simulink model "Earth_Moon"  (R2024a)
settings: Solver=VariableStepAuto  StartTime=0.0  StopTime=2419200  RelTol=1e-3
values from neighbouring files (symbols this model uses):
  G = 6.674e-11    [L_points.m]    (also in Lab3_Driver.m; Lab5.m; Lab8.m; LagrangePoints.m = 6.67408e-11)
  mE = 5.97219e24    (= 5.97219e+24)    [L_points.m]    (also in Lab5.m; Lab8.m; Presentation_Circular.m; Presentation_HaloOrbit.m)
  mM = 7.349e22    (= 7.349e+22)    [L_points.m]    (also in Lab5.m; Lab8.m; Presentation_Circular.m = plot3(OM(mid,1)/1000,OM(mid,2)/1000,OM(mid,3)/1000,Marker="o; Presentation_HaloOrbit.m)
  posE = [3.034529801433376E+03 -3.340359653273315E+03 -1.939037192252903E+03]*1000    [L_points.m]    (also in Lab5.m = [-xE 0 0]; Lab8.m = [-xE 0 0]; Presentation_Circular.m = [-xE 0 0]; Presentation_HaloOrbit.m = [-xE 0 0])
  posM = [-2.467089971416006E+05 2.715731378752839E+05 1.576448255327776E+05]*1000    [L_points.m]    (also in Lab5.m = [xM 0 0]; Lab8.m = [xM 0 0]; Presentation_Circular.m = [xM 0 0]; Presentation_HaloOrbit.m = [xM 0 0])
  velE = [9.245683416082787E-03 6.608382937807280E-03 2.954691314042687E-03]*1000    [L_points.m]    (also in Lab5.m = [0 -vE 0]; Lab8.m = [0 -vE 0]; Presentation_Circular.m = [0 -vE 0]; Presentation_HaloOrbit.m = [0 -vE 0])
  velM = [-7.516793153236040E-01 -5.372652878689789E-01 -2.402180827507927E-01]*1000    [L_points.m]    (also in Lab5.m = [0 vM 0]; Lab8.m = [0 vM 0]; Presentation_Circular.m = [0 vM 0]; Presentation_HaloOrbit.m = [0 vM 0])
settings Model: Creator=sgtjake2  LastModifiedBy=sgtjake2

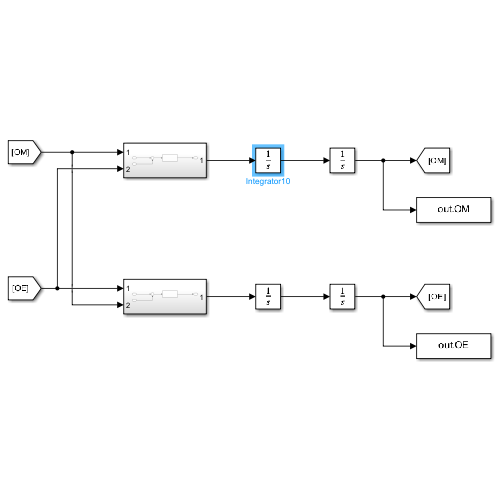
[thumbnail: Simulink's stored preview of the top-level diagram]
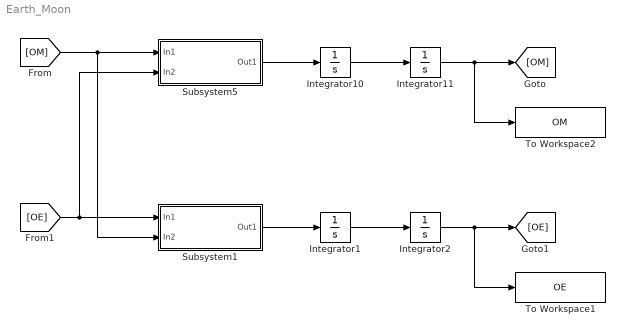
== system Earth_Moon ==
  Integrator1 : Integrator  InitialCondition=velE
  Integrator10 : Integrator  InitialCondition=velM
  Integrator11 : Integrator  InitialCondition=posM
  Integrator2 : Integrator  InitialCondition=posE
  Subsystem1 : Subsystem
  Subsystem5 : Subsystem
  To Workspace1 : ToWorkspace  VariableName=OE  SaveFormat=Timeseries  SampleTime=-1
  To Workspace2 : ToWorkspace  VariableName=OM  SaveFormat=Timeseries  SampleTime=-1
  wires:
  Integrator11/1 -> To Workspace2/1, [OM]
  [OM] -> Subsystem1/2(In2), Subsystem5/1(In1)
  Integrator10/1 -> Integrator11/1
  Integrator2/1 -> To Workspace1/1, [OE]
  [OE] -> Subsystem1/1(In1), Subsystem5/2(In2)
  Integrator1/1 -> Integrator2/1
  Subsystem5/1(Out1) -> Integrator10/1
  Subsystem1/1(Out1) -> Integrator1/1

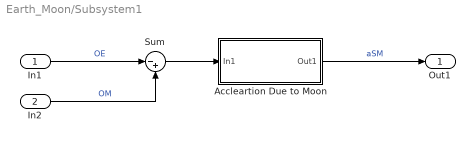
== system Earth_Moon/Subsystem1 ==
  In1 : Inport
  In2 : Inport  Port=2
  Accleartion Due to Moon : Subsystem
  Sum : Sum  Inputs=|-+
  Out1 : Outport
  wires:
  Accleartion Due to Moon/1(Out1) -> Out1/1  "aSM"
  Sum/1 -> Accleartion Due to Moon/1(In1)
  In1/1 -> Sum/1  "OE"
  In2/1 -> Sum/2  "OM"

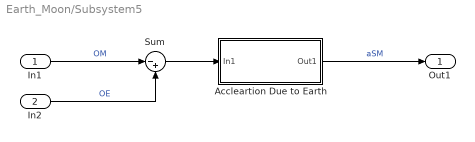
== system Earth_Moon/Subsystem5 ==
  In1 : Inport
  In2 : Inport  Port=2
  Accleartion Due to Earth : Subsystem
  Sum : Sum  Inputs=|-+
  Out1 : Outport
  wires:
  Accleartion Due to Earth/1(Out1) -> Out1/1  "aSM"
  Sum/1 -> Accleartion Due to Earth/1(In1)
  In1/1 -> Sum/1  "OM"
  In2/1 -> Sum/2  "OE"

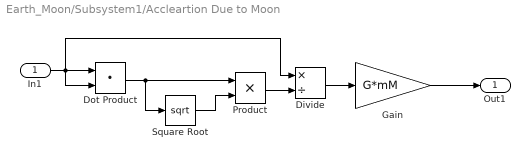
== system Earth_Moon/Subsystem1/Accleartion Due to Moon ==
  In1 : Inport
  Divide : Product  Inputs=*/
  Dot Product : DotProduct  OutDataTypeStr=Inherit: Inherit via internal rule
  Gain : Gain  Gain=G*mM
  Product : Product
  Square Root : Sqrt
  Out1 : Outport
  wires:
  In1/1 -> Divide/1, Dot Product/2, Dot Product/1
  Dot Product/1 -> Square Root/1, Product/1
  Square Root/1 -> Product/2
  Product/1 -> Divide/2
  Gain/1 -> Out1/1
  Divide/1 -> Gain/1

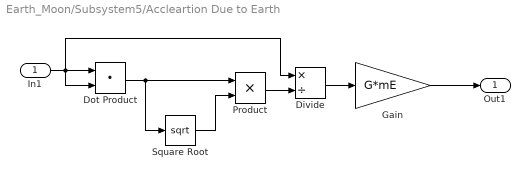
== system Earth_Moon/Subsystem5/Accleartion Due to Earth ==
  In1 : Inport
  Divide : Product  Inputs=*/
  Dot Product : DotProduct  OutDataTypeStr=Inherit: Inherit via internal rule
  Gain : Gain  Gain=G*mE
  Product : Product
  Square Root : Sqrt
  Out1 : Outport
  wires:
  In1/1 -> Divide/1, Dot Product/2, Dot Product/1
  Dot Product/1 -> Square Root/1, Product/1
  Square Root/1 -> Product/2
  Product/1 -> Divide/2
  Gain/1 -> Out1/1
  Divide/1 -> Gain/1
